simulink model "Torque_Vectoring_Controller_Controls_2018_Test"  (R2017b)
settings: Solver=ode45  StartTime=0.0  StopTime=inf  RelTol=1e-3  EnableMultiTasking=on
InitFcn:
  | clear_close
  | dataCar
  | optParam
  | structSensors
  | structSettings
  | structEstimPar
  | structAero
  | structVariables
  | readFuzzyFile
StartFcn:
  | clear_close
  | dataCar
  | optParam
  | structSensors
  | structSettings
  | structEstimPar
  | structAero
  | structVariables
  | readFuzzyFile
undefined symbols (not defined in the file or in its folder): car, sensors
libraries: CarMaker4SL x21, simulink x11
(part 3 of 4)

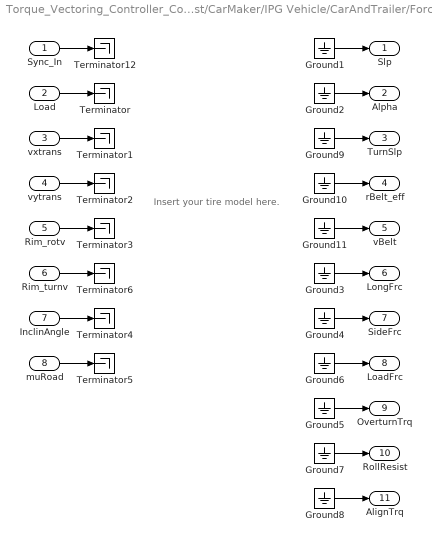
== system Torque_Vectoring_Controller_Controls_2018_Test/CarMaker/IPG Vehicle/CarAndTrailer/Forces/Tires/TireRL ==
  note: Insert your tire model here.
  Sync_In : Inport
  Load : Inport  Port=2
  vxtrans : Inport  Port=3
  vytrans : Inport  Port=4
  Rim_rotv : Inport  Port=5
  Rim_turnv : Inport  Port=6
  InclinAngle : Inport  Port=7
  muRoad : Inport  Port=8
  Ground{1..11} (11 alike) : Ground
  Terminator{,1..6,12} (8 alike) : Terminator
  Slp : Outport
  Alpha : Outport  Port=2
  TurnSlp : Outport  Port=3
  rBelt_eff : Outport  Port=4
  vBelt : Outport  Port=5
  LongFrc : Outport  Port=6
  SideFrc : Outport  Port=7
  LoadFrc : Outport  Port=8
  OverturnTrq : Outport  Port=9
  RollResist : Outport  Port=10
  AlignTrq : Outport  Port=11
  wires:
  Ground11/1 -> vBelt/1
  Ground10/1 -> rBelt_eff/1
  Ground9/1 -> TurnSlp/1
  Rim_turnv/1 -> Terminator6/1
  Sync_In/1 -> Terminator12/1
  Ground2/1 -> Alpha/1
  Ground3/1 -> LongFrc/1
  Ground4/1 -> SideFrc/1
  Ground5/1 -> OverturnTrq/1
  vxtrans/1 -> Terminator1/1
  vytrans/1 -> Terminator2/1
  Rim_rotv/1 -> Terminator3/1
  InclinAngle/1 -> Terminator4/1
  muRoad/1 -> Terminator5/1
  Load/1 -> Terminator/1
  Ground1/1 -> Slp/1
  Ground6/1 -> LoadFrc/1
  Ground7/1 -> RollResist/1
  Ground8/1 -> AlignTrq/1

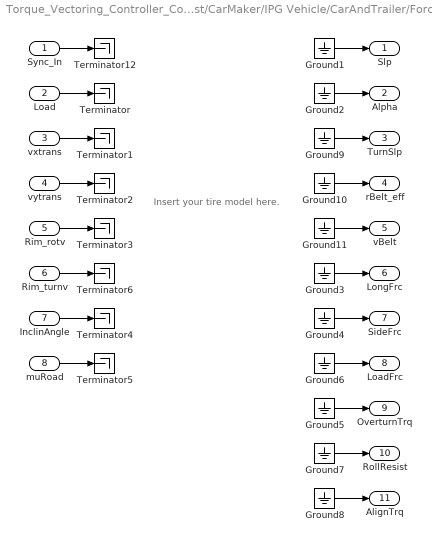
== system Torque_Vectoring_Controller_Controls_2018_Test/CarMaker/IPG Vehicle/CarAndTrailer/Forces/Tires/TireRR ==
  note: Insert your tire model here.
  Sync_In : Inport
  Load : Inport  Port=2
  vxtrans : Inport  Port=3
  vytrans : Inport  Port=4
  Rim_rotv : Inport  Port=5
  Rim_turnv : Inport  Port=6
  InclinAngle : Inport  Port=7
  muRoad : Inport  Port=8
  Ground{1..11} (11 alike) : Ground
  Terminator{,1..6,12} (8 alike) : Terminator
  Slp : Outport
  Alpha : Outport  Port=2
  TurnSlp : Outport  Port=3
  rBelt_eff : Outport  Port=4
  vBelt : Outport  Port=5
  LongFrc : Outport  Port=6
  SideFrc : Outport  Port=7
  LoadFrc : Outport  Port=8
  OverturnTrq : Outport  Port=9
  RollResist : Outport  Port=10
  AlignTrq : Outport  Port=11
  wires:
  Ground11/1 -> vBelt/1
  Ground10/1 -> rBelt_eff/1
  Ground9/1 -> TurnSlp/1
  Rim_turnv/1 -> Terminator6/1
  Sync_In/1 -> Terminator12/1
  Ground2/1 -> Alpha/1
  Ground3/1 -> LongFrc/1
  Ground4/1 -> SideFrc/1
  Ground5/1 -> OverturnTrq/1
  vxtrans/1 -> Terminator1/1
  vytrans/1 -> Terminator2/1
  Rim_rotv/1 -> Terminator3/1
  InclinAngle/1 -> Terminator4/1
  muRoad/1 -> Terminator5/1
  Load/1 -> Terminator/1
  Ground1/1 -> Slp/1
  Ground6/1 -> LoadFrc/1
  Ground7/1 -> RollResist/1
  Ground8/1 -> AlignTrq/1

== matlab function Torque_Vectoring_Controller_Controls_2018_Test/CarMaker/Controls/Control Systems/Traction Control ==
  data: sensors input; Torques output; settings input; estimPar input; torqueDistribution input; slipSet input; car parameter; TiTi2 output; error output; rpmSet output
function [Torques, TiTi2, error, rpmSet] = Traction(sensors, settings, estimPar, torqueDistribution, slipSet, car)

Torquesmin = -car.motor.Tmax;
Torquesmax = car.motor.Tmax;
rpmSetmin = -20000;
rpmSetmax = 20000;

error =[0 0 0 0]';
persistent errorInt; if isempty(errorInt); errorInt=[0 0 0 0]'; end
persistent errorD; if isempty(errorD); errorD=[0 0 0 0]'; end
persistent errorPrev; if isempty(errorPrev); errorPrev=[0 0 0 0]'; end

%persistent wi_prev; if isempty(wi_prev); wi_prev=[0 0 0 0]'; end
%persistent SR_expected; if isempty(SR_expected); SR_expected=zeros(4, 8); end
%persistent wvi_prev; if isempty(wvi_prev); wvi_prev=[0 0 0 0]'; end

persistent TiPrev; if isempty(TiPrev); TiPrev=[0 0 0 0]'; end

persistent errorInt2; if isempty(errorInt2); errorInt2=[0 0 0 0]'; end
persistent Ti; if isempty(Ti); Ti=[0 0 0 0]'; end
persistent Ti2; if isempty(Ti2); Ti2=[0 0 0 0]'; end

rpmSet = [20000;20000;20000;20000];

if settings.TC == 1

    slipRatioTarget = slipSet;
    dist = estimPar.Fzi/sum(estimPar.Fzi);
    
    Kp = 1000*dist*10;
    Ki = 40*dist*1000;
    Kd = 0*dist/100;
    Kv = 1;
    Mu = 1.40;
    
    Kp2 = 20*dist/1000;
    Ki2 = 40*dist/1000;
    
    %normal non linear torque control
    error = slipRatioTarget - estimPar.slip;
    
    errorInt = errorInt + error*car.dt;
    errorInt = min(max(errorInt,-0.001*[1;1;1;1]),0.003*[1;1;1;1]);
    errorD = min(max(errorD*0.1 + 0.9*(error - errorPrev)/car.dt,-25),25);
    lambdaD = Kp.*error + Ki.*errorInt + Kd.*errorD;
    Ti = lambdaD*car.tireInertia*max(estimPar.v,0)^Kv/car.tireRadius + sign(torqueDistribution).*estimPar.Fzi*(Mu)*car.tireRadius;
    Ti = Ti / car.gearRatio;
    
    %optimum seeking
    dFds = dFdsCalculator(estimPar.Fxi,estimPar.slip);
    error2 = dFds - 0;
    errorInt2 = errorInt2 + error2*car.dt;
    errorInt2 = min(max(errorInt2,-500*[1;1;1;1]),500*[1;1;1;1]);
    lambdaD2 = Kp2.*error2 + Ki2.*errorInt2;
    Ti2 = lambdaD2*car.tireInertia*max(estimPar.v,0)^Kv/car.tireRadius + sign(torqueDistribution).*estimPar.Fzi*(car.TC_mu)*car.tireRadius;
    Ti2 = Ti2 / car.gearRatio;
    
    for i=1:4
        if abs(error(i)) < 0.05
            Ti(i) = Ti2(i);
        end
    end
    
    if estimPar.v < 1/3.6
        %Ti = [80 80 180 180]';
        errorInt = [0 0 0 0]';
    end

    if sensors.throttle < 0.1
        errorInt = [0 0 0 0]';
    end
    
    lowerBoundary = TiPrev - 100/car.gearRatio;
    upperBoundary = TiPrev + 100/car.gearRatio;

    Ti = min(max(Ti,lowerBoundary),upperBoundary);
    
    TiPrev = Ti;
    errorPrev = error;
    
    Torques = Ti;
    for i=1:4
        if torqueDistribution(i) > 0
            Torques(i) = max(min(Torques(i),torqueDistribution(i)),0); 
        else
            Torques(i) = min(max(Torques(i),torqueDistribution(i)),0);
        end
    end
    
    
else
    Torques = torqueDistribution;
end

checkTorquemax = find((Torques > car.motor.Tmax)==1); %Limit torques to max torque
Torques(checkTorquemax)=car.motor.Tmax(checkTorquemax);



%wi_prev = sensors.wheelspeed;
%wvi_prev = sensors.wheelspeedi;

TiTi2 = [Ti;Ti2];

Torques = min(max(Torques,Torquesmin),Torquesmax);
rpmSet = min(max(rpmSet,rpmSetmin),rpmSetmax);

end

function [dFds] = dFdsCalculator(Fx,slipRatio)
N = 6;

persistent slipVector, if isempty(slipVector); slipVector = zeros(N,4); end
persistent FxVector, if isempty(FxVector); FxVector = zeros(N,4); end


FxVector(1,:) = Fx;
slipVector(1,:) = slipRatio;

dFds = [0;0;0;0];

for i=1:4
    p1 = polyfit(slipVector(:,i),FxVector(:,i),1);
    p2 = polyfit(FxVector(:,i),slipVector(:,i),1);
    
    rico1 = p1(1);
    rico2 = 1/p2(1);
    
    rico = sign(min(abs(rico1),abs(rico2)))*min(abs(rico1),abs(rico2));

    dFds(i) = max(min(rico,20000),-20000);
end

% shift list one
dummy = FxVector(1:N-1,:);
FxVector = [[0,0,0,0];dummy];
dummy = slipVector(1:N-1,:);
slipVector = [[0,0,0,0];dummy];


end

== matlab function Torque_Vectoring_Controller_Controls_2018_Test/CarMaker/Controls/Vehicle Estimated Parameters/Global model calculation ==
  data: sensors input; F_KF output; States input; H_KF output; y_pred output; yawrate_lin output; beta_lin output; car parameter
function [F_KF, H_KF, y_pred, yawrate_lin, beta_lin] = global_model(sensors, States, car)

global vy_g psi_dot_g vx_g Cf_g Cr_g vy_lin psi_dot_lin

if isempty(vy_g) == 1 && isempty(psi_dot_g) == 1 && isempty(vx_g) == 1 ...
        && isempty(Cf_g) == 1 && isempty(Cr_g) == 1 
    States.vy_g = 0;
    States.psi_dot_g = 0;
    States.vx_g = 0;
    States.Cf_g = 0;
    States.Cr_g = 0;
    
else 
    
    States.vy_g = vy_g;
    States.psi_dot_g = psi_dot_g;
    States.vx_g = vx_g;
    States.Cf_g = Cf_g;
    States.Cr_g = Cr_g;
    delta = (sensors.wheelAngles(1)+sensors.wheelAngles(2))/2;
    
    %% Calculating F_KF %%
    
    F_vy = [-(2*(States.Cf_g+States.Cr_g))/(car.mass*States.vx_g),...
        -((2*(States.Cf_g*car.lf-States.Cr_g*car.lr))/(car.mass*States.vx_g))+States.vx_g,...
        (((2*(States.Cf_g+States.Cr_g))/(car.mass*States.vx_g^2))*States.vy_g)+...
        (((2*(States.Cf_g*car.lf-States.Cr_g*car.lr))/(car.mass*States.vx_g^2))*States.psi_dot_g)-States.psi_dot_g,...
        (-2/(car.mass*States.vx_g))*(States.vy_g+car.lf*States.psi_dot_g)+(2*delta/car.mass),...
        (-2/(car.mass*States.vx_g))*(States.vy_g-car.lr*States.psi_dot_g)];
    
    F_psi_dot = [-(2*(States.Cf_g*car.lf-States.Cr_g*car.lr))/(car.yawInertia*States.vx_g),...
        -((2*(States.Cf_g*car.lf^2+States.Cr_g*car.lr^2))/(car.yawInertia*States.vx_g)),...
        (((2*(States.Cf_g*car.lf-States.Cr_g*car.lr))/(car.yawInertia*States.vx_g^2))*States.vy_g)+...
        (((2*(States.Cf_g*car.lf^2+States.Cr_g*car.lr^2))/(car.yawInertia*States.vx_g^2))*States.psi_dot_g),...
        (-2*car.lf/(car.yawInertia*States.vx_g))*(States.vy_g+car.lf*States.psi_dot_g)+(2*delta*car.lf/car.yawInertia),...
        (2*car.lr/(car.yawInertia*States.vx_g))*(States.vy_g-car.lr*States.psi_dot_g)];
    
    F_vx = [States.psi_dot_g, States.vy_g,0,0,0];
    
    F_Cf = [0,0,0,0,0];
    
    F_Cr = [0,0,0,0,0];
    
    F_KF = [F_vy;F_psi_dot;F_vx;F_Cf;F_Cr];
    
    %% Calculation vy_lin and beta_lin %% Gelineariseerd, hier kan eventueel ook
    % ode45 voor gebruikt worden.
    
   A_1 = (-2*(car.Cf_lin + car.Cr_lin))/(car.mass*States.vx_g);
   A_2 = -((2*(car.Cf_lin*car.lf - car.Cr_lin*car.lr))/(car.mass*States.vx_g))+States.vx_g;
   A_3 = -(2*(car.Cf_lin*car.lf - car.Cr_lin*car.lr))/(car.yawInertia*States.vx_g);
   A_4 = (-2*(car.Cf_lin*car.lf^2 + car.Cr_lin*car.lr^2))/(car.yawInertia*States.vx_g);
   
   B_1 = (2*car.Cf_lin*delta)/(car.mass);
   B_2 = (2*car.Cf_lin*car.lf*delta)/(car.yawInertia);
      
   A = [1+A_1*car.dt, A_2*car.dt; A_3*car.dt 1+A_4*car.dt];
   B = [B_1; B_2];
   
   
   lin_var = A*[vy_lin;psi_dot_lin] + B;
   vy_lin = lin_var(1);
   psi_dot_lin = lin_var(2);
   yawrate_lin =  psi_dot_lin;
   beta_lin = vy_lin/(States.vx);
    
    %% Calculation H_KF %%
    
    H_psi_dot = [0, 1, 0, 0,0];
    
    H_ay = [-(2*(States.Cf_g+States.Cr_g))/(car.mass*States.vx_g),...
        -((2*(States.Cf_g*car.lf-States.Cr_g*car.lr))/(car.mass*States.vx_g)),...
        (((2*(States.Cf_g+States.Cr_g))/(car.mass*States.vx_g^2))*States.vy_g)+...
        (((2*(States.Cf_g*car.lf-States.Cr_g*car.lr))/(car.mass*States.vx_g^2))*States.psi_dot_g),...
        (-2/(car.mass*States.vx_g))*(States.vy_g+car.lf*States.psi_dot_g)+(2*delta/car.mass),...
        (-2/(car.mass*States.vx_g))*(States.vy_g-car.lr*States.psi_dot_g)];
    
    H_vxfl = [sin(sensors.wheelAngles(1)),  -(car.tf/2)*cos(sensors.wheelAngles(1))+car.lf*sin(sensors.wheelAngles(1)), cos(sensors.wheelAngles(1)), 0, 0];
    
    H_vxfr = [sin(sensors.wheelAngles(2)), (car.tf/2)*cos(sensors.wheelAngles(2))+car.lf*sin(sensors.wheelAngles(2)), cos(sensors.wheelAngles(2)),  0, 0];
    
    H_vxrl = [0, -(car.tr/2), 1, 0, 0];
    
    H_vxrr = [0, (car.tr/2), 1, 0, 0];
    
    H_beta_lin = [0,0,-(vy_lin/States.vx_g^2),0,0]; %afgeleide naar vx herplaatst, die naar vy = 0?
    
    H_KF = [H_psi_dot;H_ay;H_vxfl;H_vxfr;H_vxrl;H_vxrr; H_beta_lin];

    %% Calculation of y_pred
    
    y_pred.yawrate = States.psi_dot_g;
    
    y_pred.ay = (-2*(States.Cf_g+States.Cr_g)/(car.mass*States.vx_g))*(States.vy) - ...
        (2*(States.Cf_g*car.lf-States.Cr_g*car.lr)/(car.mass*States.vx_g))*(States.psi_dot_g) +... % - teken aangepast naar vgl (7) uit van Aalst
        (2*States.Cf_g*delta/car.mass);
    
    y_pred.vxfl = (States.vx_g - States.psi_dot_g*(car.tf/2))*cos(sensors.wheelAngles(1)) + ...
        (States.vy_g + States.psi_dot_g*(car.lf))*sin(sensors.wheelAngles(1));
    
    y_pred.vxfr = (States.vx_g + States.psi_dot_g*(car.tf/2))*cos(sensors.wheelAngles(2)) + ...
        (States.vy_g + States.psi_dot_g*(car.lf))*sin(sensors.wheelAngles(2));
    
    y_pred.vxrl = (States.vx_g - States.psi_dot_g*(car.tr/2));
    
    y_pred.vxrr = (States.vx_g + States.psi_dot_g*(car.tr/2));
    
    y_pred.beta_lin = (vy_lin)/(States.vx);
    
end
end

== matlab function Torque_Vectoring_Controller_Controls_2018_Test/CarMaker/Controls/Control Systems/Yaw Rate Control ==
  data: sensors input; Mz output; settings input; estimPar input; car parameter; error output; actions output; rref output
function [Mz,error,actions,rref]= yawRateControl(sensors, settings, estimPar, car)
%Function that controls the moment around the z-axis
%INPUTS:
%OUTPUT: Moment of the car around Z-axis [Nm]

Mz = 0;
Mz_temp = 0;
rref = estimPar.rref;
error = 0;


wheelAngle = (sensors.wheelAngles(1)+sensors.wheelAngles(2))/2;

%For analyzation
P_Action = 0;
I_Action = 0;
D_Action = 0;

steeringWheel_Action = 0;
yawRate_Action = 0;

persistent Mz_memory; if isempty(Mz_memory); Mz_memory = 0; end
persistent errorInt; if isempty(errorInt); errorInt = 0; end
persistent errorDev; if isempty(errorDev); errorDev = 0; end
persistent prevError; if isempty(prevError); prevError = 0; end
persistent prevWheelAngle; if isempty(prevWheelAngle); prevWheelAngle = 0; end
persistent prevRref; if isempty(prevRref); prevRref = 0; end

%if settings.YRCMode == 1
error = estimPar.rref - sensors.yawRate;
errorInt = errorInt + error*car.dt;
errorInt = min(max(errorInt,-car.YRC.intLimit),car.YRC.intLimit);
errorDev = (error - prevError)/car.dt;
wheelAngleFF = wheelAngle;


velocityGain = min(max(1 - (estimPar.v - car.YRC.changeVelocity)*car.YRC.slope,0),1);

Mz_temp = (car.YRC.Kp*error + car.YRC.Ki*errorInt + car.YRC.Kd*errorDev...
    +car.YRC.Ks*wheelAngleFF)*velocityGain;
Mz_temp = max(min(Mz_temp,car.YRC.maxValue),-car.YRC.maxValue);
Mz_memory=Mz_memory+Mz_temp;

P_Action = car.YRC.Kp*error;
I_Action = car.YRC.Ki*errorInt;
D_Action = car.YRC.Kd*errorDev;
steeringWheel_Action = car.YRC.Ks*wheelAngle;
yawRate_Action = car.YRC.Kr*estimPar.rref;

actions = [P_Action;I_Action;D_Action;steeringWheel_Action;yawRate_Action];
prevError = error;
prevWheelAngle = wheelAngle;
prevRref = estimPar.rref;
%end


% if settings.YRCMode == 2
%     error = estimPar.rref - sensors.yawRate;
%     integral = integral + error*car.dt;
%     derivative = (error - prevError)/car.dt;
%
%     Mz_temp = car.YRC.Kp*error + car.YRC.Ki*integral + car.YRC.Kd*derivative...
%         +car.YRC.Ks*wheelAngle + car.YRC.Kr*estimPar.rref;
%     Mz_temp = max(min(Mz_temp,car.YRC.maxValue),-car.YRC.maxValue);
%
%     prevError = error;
% end





%YRC enabled
if settings.YRC ==1
    Mz = Mz_memory;
    
    %YRC disabled
else
    Mz = 0;
end

if car.YRC.minV > estimPar.v
    Mz = 0; %if speed is too low, don't activate yaw rate control
    errorInt = 0;
    prevError = 0;
end



rref=estimPar.rref;

Mz = min(max(Mz,-car.MzMax),car.MzMax); % set limits to maximum sent out Mz

== matlab function Torque_Vectoring_Controller_Controls_2018_Test/CarMaker/Controls/Controller Settings/Controller Settings ==
  data: settings output Bus: settingBus; sensors input; variables output Bus: variableBus
function [settings,variables] = settingController(sensors)

%% Settings

%Afblijven van dit, dit is de default instelling
velocityEstimation_Temp = 0;
YRCMode_Temp = 0;
torqueMode_Temp = 0;
YRC_Temp = 0;
TC_Temp = 0;
unlimitedFx_Temp = 0;
effEstimation_Temp = 0;


%if sensors.knob1 == 1
    YRC_Temp = 1;
%end

%if sensors.knob1 == 1
    torqueMode_Temp = 2; %Change distributor mode
%end

%if sensors.knob2 == 1
    YRCMode_Temp = 1;
    TC_Temp = 0;
    unlimitedFx_Temp = 0;
    TV_bypass_Temp = 0;
%end
velocityEstimation_Temp = 1;
%if sensors.knob2 == 2
    %YRCMode_Temp = 2;
%end

effEstimation_Temp = 2;

%% Variables
TD_percentage_Temp = 1;


%% Declaration Settings

settings.velocityEstimation = velocityEstimation_Temp;
settings.torqueMode = torqueMode_Temp;
settings.YRC = YRC_Temp;
settings.YRCMode = YRCMode_Temp;
settings.distributorMode = 0;

settings.Fsens = 100; %value between 0 and 100
% 100 --> Fdes is really important
% 0 --> Mdes is really important

settings.Fxsens = 1;

settings.TC = TC_Temp;
settings.unlimitedFx = unlimitedFx_Temp;
settings.TV_bypass = TV_bypass_Temp;
settings.effEstimation = effEstimation_Temp;

%% Declaration Variables
variables.TD_percentage = TD_percentage_Temp;

== matlab function Torque_Vectoring_Controller_Controls_2018_Test/CarMaker/Controls/Vehicle Estimated Parameters/Scopes/States decomposition ==
  data: States input; vy output; psi_dot output; vx output; Cf output; Cr output
function [vy,psi_dot,vx,Cf,Cr] = state_decomp(States)

vy = States.vy_g;
psi_dot = States.psi_dot_g;
vx = States.vx_g;
Cf = States.Cf_g;
Cr = States.Cr_g;

== matlab function Torque_Vectoring_Controller_Controls_2018_Test/CarMaker/Controls/Vehicle Estimated Parameters/Scopes/alpha decomposition ==
  data: alpha input; alpha_f output; alpha_r output
function [alpha_f, alpha_r] = alpha_decomp(alpha)

alpha_f = alpha.f;
alpha_r = alpha.r;

end

== matlab function Torque_Vectoring_Controller_Controls_2018_Test/CarMaker/Controls/Vehicle Estimated Parameters/Velocity and alpha decomposition ==
  data: States input; vx_wheels output; vy_wheels output; alpha_wheels output; sensors parameter; car parameter
function [vx_wheels, vy_wheels, alpha_wheels] = v_alpha_decomp(States, sensors, car)

%% Calculation vx on each independant wheel %%

vx_wheels.fl = (States.vx_g - States.psi_dot_g*(car.tf/2))*cos(sensors.wheelAngles(1)) + ...
        States.psi_dot_g*(car.lf)*sin(sensors.wheelAngles(1));
    
vx_wheels.fr = (States.vx_g + States.psi_dot_g*(car.tf/2))*cos(sensors.wheelAngles(2)) + ...
        States.psi_dot_g*(car.lf)*sin(sensors.wheelAngles(2));
    
vx_wheels.rl = (States.vx_g - States.psi_dot_g*(car.tr/2));
    
vx_wheels.rr = (States.vx_g + States.psi_dot_g*(car.tr/2));

%% Calculation vy on each independant wheel %%

vy_wheels.fl = (States.vy_g + States.psi_dot_g*(car.lf))*cos(sensors.wheelAngles(1)) + ...
        States.psi_dot_g*(car.tf/2)*sin(sensors.wheelAngles(1));
    
vy_wheels.fr = (States.vy_g - States.psi_dot_g*(car.tf/2))*sin(sensors.wheelAngles(2)) + ...
        States.psi_dot_g*(car.lf)*cos(sensors.wheelAngles(2));
    
vy_wheels.rl = (States.vy_g - States.psi_dot_g*(car.lr));
    
vy_wheels.rr = (States.vy_g - States.psi_dot_g*(car.lr));

%% Calculation alpha's on each independant wheel %%

alpha_wheels.fl = atan2(vy_wheels.fl,vx_wheels.fl);
alpha_wheels.fr = atan2(vy_wheels.fr,vx_wheels.fr);
alpha_wheels.rl = atan2(vy_wheels.rl,vx_wheels.rl);
alpha_wheels.rr = atan2(vy_wheels.rr,vx_wheels.rr);

== matlab function Torque_Vectoring_Controller_Controls_2018_Test/CarMaker/Controls/Control Systems/Distributor/MATLAB Function ==
  data: sensors input; torqueDistribution output; settings input; estimPar input; car parameter; variables input; Mz input; slipSet output; Fdes output; sumFx output; Fxmax output; Fxmaxsum output; Fx output; Fdes input
function [torqueDistribution, slipSet,Fdes,sumFx,Fxmax,Fxmaxsum, Fx]= TorqueDistributor(sensors,settings, estimPar, car, variables, Mz, Fdes)
%,Fdes,sumFx,Fxmax,Fxmaxsum

torqueDistribution = [0;0;0;0];
slipSet = [0;0;0;0];


sumFx=0;
Fxmax=[0;0;0;0];
Fxmaxsum=0;
Fx=[0;0;0;0];
if settings.torqueMode == 1
    
    dT =  0.25*Mz/(car.tw*0.5)*car.tireRadius;
    torqueDistribution = car.motor.Tmax*variables.TD_percentage*sensors.throttle;
    torqueDistribution = torqueDistribution + [-1; 1; -1; 1]*dT;
    
    for i=1:4
        if torqueDistribution(i) > 0
            slipSet(i) = car.TC.slipSetAcc;
        else
            slipSet(i) = car.TC.slipSetBrake;
        end
    end
    
    
end



%Test torque mode: only Fx, no steeringAngle

if settings.torqueMode == 2
    

    
    Fxmax = [0;0;0;0];
    %minForce = 2*car.Cd*car.AFront*0.5*car.rhoAir*estimPar.v*estimPar.v*0.25; %2* of niet? en met Cd?
    minForce = 0;
    %FyReduceFactor = 0.1;
    %Fxmax = (max((estimPar.mu .* estimPar.Fzi).^2-FyReduceFactor*estimPar.Fyi.^2,0).^0.5); %Kamm's circle
    
    
    
    Fxmax = estimPar.mu.*estimPar.Fzi;
    
    Fxmax = max(Fxmax,minForce);
    motorSpeed = min(max(sensors.wheelspeed.*car.gearRatio,0),20000);
    FxmaxMax = [car.FxmaxMax(round(motorSpeed(1)+1));...
        car.FxmaxMax(round(motorSpeed(2)+1));...
        car.FxmaxMax(round(motorSpeed(3)+1));...
        car.FxmaxMax(round(motorSpeed(4)+1))];  %make sure the max torque of the motor isn't surpassed

%     x = 0:10:22000; y = [0 .15 1.12 2.36 2.36 1.46 .49 .06 0];
%     cs = spline(x,[0 y 0]);
%     xx = linspace(-4,4,101);
%     plot(x,y,'o',xx,ppval(cs,xx),'-');
    
    checkFxmax = find((Fxmax > FxmaxMax)==1);
    Fxmax(checkFxmax)=FxmaxMax(checkFxmax);
    
    if settings.unlimitedFx == 1  %Surpass the tire grip limits in case if the driver feels to restricted with this.
        Fxmax = FxmaxMax;
    end
    
    Fxmaxsum = sum(Fxmax);
    Fxmin = -Fxmax;
    
    Fx = [0;0;0;0];
    
    
    Fx = Distributor(settings, car, Mz, Fdes, Fxmax, Fxmin);
    
    torqueDistribution = car.tireRadius*Fx; %torque of motor, NOT of wheels (as IPG expects this as input)
    
    for i=1:4
        if torqueDistribution(i) > 0
            slipSet(i) = car.TC.slipSetAcc;
        else
            slipSet(i) = car.TC.slipSetBrake;
        end
    end
    
    sumFx = sum(Fx);
end



torqueDistribution = min(max(torqueDistribution,-car.motor.Tmax),car.motor.Tmax); % dees nog ifv motorkarakteristiek
end

== matlab function Torque_Vectoring_Controller_Controls_2018_Test/CarMaker/Controls/Bypass/MATLAB Function ==
  data: settings input; torqueBypass output; sensors input; rpmBypass output; car parameter
function [torqueBypass,rpmBypass]= fcn(settings, sensors, car)
PmaxTyre = car.Pmax_bypass*0.25;
rad2rpm = 30/pi;


safetyFactor = 0.5;
torqueBypass = car.motor.Tmax*safetyFactor*car.gearRatio*sensors.throttle;

if sensors.throttle > 0
    rpmBypass = car.motor.rpmMax;
else
    rpmBypass = [0;0;0;0];
end

%% Power limiter
limit = PmaxTyre./max(sensors.wheelspeed,1);
torqueBypass = max(min(torqueBypass,limit),-limit);

== matlab function Torque_Vectoring_Controller_Controls_2018_Test/CarMaker/Controls/Vehicle Estimated Parameters/Scopes/Longitudinal velocity decomposition ==
  data: vx_wheels input; vx_fl output; vx_fr output; vx_rl output; vx_rr output
function [vx_fl, vx_fr, vx_rl, vx_rr] = long_vel_decomp(vx_wheels)

vx_fl = vx_wheels.fl;
vx_fr = vx_wheels.fr;
vx_rl = vx_wheels.rl;
vx_rr = vx_wheels.rr;

end

== matlab function Torque_Vectoring_Controller_Controls_2018_Test/CarMaker/Controls/Tire model//friction coefficient estimation/MATLAB Function ==
  data: mu input; estimParExtended output; estimPar input
function estimParExtended  = estimParExtension(mu, estimPar)

estimParExtended.vy_g = estimPar.vy_g;
estimParExtended.psi_dot_g = estimPar.psi_dot_g;
estimParExtended.vx_g = estimPar.vx_g;
estimParExtended.Cf_g = estimPar.Cf_g;
estimParExtended.Cr_g = estimPar.Cr_g;
estimParExtended.Fzi=estimPar.Fzi;
estimParExtended.Fxi=estimPar.Fxi;
estimParExtended.Fyi=estimPar.Fyi;
estimParExtended.alpha_f = estimPar.alpha.f;
estimParExtended.alpha_r = estimPar.alpha.r;
estimParExtended.eff = estimPar.eff;
estimParExtended.mu = mu;
estimParExtended.rref = estimPar.rref;

== matlab function Torque_Vectoring_Controller_Controls_2018_Test/CarMaker/IPG Feedback/Subsystem/MATLAB Function ==
  data: Wheelspeed_Max input; T_mot output; Wheelspeed_Sens input; Treq input
function T_mot = SpeedLimit(Wheelspeed_Max,Wheelspeed_Sens,Treq)
%Speed limiter for IPG Carmaker
if Wheelspeed_Sens>= Wheelspeed_Max
    T_mot=0;
else
    T_mot=Treq;
end

== matlab function Torque_Vectoring_Controller_Controls_2018_Test/CarMaker/Controls/Tire model//friction coefficient estimation/Magic_Tire_Param_Scope ==
  data: Magic_tire_param input; MTF_tire_model_front_x output; estimParBus input; Fzi input; MTF_tire_model_front_y output; MTF_tire_model_rear_x output; MTF_tire_model_rear_y output
function [MTF_tire_model_front_x, MTF_tire_model_front_y,MTF_tire_model_rear_x,...
    MTF_tire_model_rear_y] = Scope_Magig_tire(Magic_tire_param, estimParBus, Fzi)

MTF_tire_model_front_x = (Fzi(1)*Magic_tire_param.front_x(3))*sin(Magic_tire_param.front_x(2)*...
    atan(Magic_tire_param.front_x(1)*(1-Magic_tire_param.front_x(4))*estimParBus.alpha_f +...
    atan(Magic_tire_param.front_x(1)*estimParBus.alpha_f)));

MTF_tire_model_front_y = (Fzi(2)*Magic_tire_param.front_y(3))*sin(Magic_tire_param.front_y(2)*...
    atan(Magic_tire_param.front_y(1)*(1-Magic_tire_param.front_y(4))*estimParBus.alpha_r +...
    atan(Magic_tire_param.front_y(1)*estimParBus.alpha_r)));

MTF_tire_model_rear_x = (Fzi(3)*Magic_tire_param.rear_x(3))*sin(Magic_tire_param.rear_x(2)*...
    atan(Magic_tire_param.rear_x(1)*(1-Magic_tire_param.rear_x(4))*estimParBus.alpha_f +...
    atan(Magic_tire_param.rear_x(1)*estimParBus.alpha_f)));

MTF_tire_model_rear_y = (Fzi(4)*Magic_tire_param.rear_y(3))*sin(Magic_tire_param.rear_y(2)*...
    atan(Magic_tire_param.rear_y(1)*(1-Magic_tire_param.rear_y(4))*estimParBus.alpha_r +...
    atan(Magic_tire_param.rear_y(1)*estimParBus.alpha_r)));

end

== matlab function Torque_Vectoring_Controller_Controls_2018_Test/CarMaker/Controls/Vehicle Estimated Parameters/Scopes/Lateral velocity decomposition1 ==
  data: vy_wheels input; vy_fl output; vy_fr output; vy_rl output; vy_rr output
function [vy_fl, vy_fr, vy_rl, vy_rr] = lat_vel_decomp(vy_wheels)

vy_fl = vy_wheels.fl;
vy_fr = vy_wheels.fr;
vy_rl = vy_wheels.rl;
vy_rr = vy_wheels.rr;

end

== matlab function Torque_Vectoring_Controller_Controls_2018_Test/CarMaker/Controls/Vehicle Estimated Parameters/Scopes/Slip angle decomposition1 ==
  data: alpha_wheels input; alpha_fl output; alpha_fr output; alpha_rl output; alpha_rr output
function [alpha_fl, alpha_fr, alpha_rl, alpha_rr] = alpha_decomp(alpha_wheels)

alpha_fl = alpha_wheels.fl;
alpha_fr = alpha_wheels.fr;
alpha_rl = alpha_wheels.rl;
alpha_rr = alpha_wheels.rr;

end

== matlab function Torque_Vectoring_Controller_Controls_2018_Test/CarMaker/IPG Feedback/Subsystem/MATLAB Function1 ==
  data: Wheelspeed_Max input; T_mot output; Wheelspeed_Sens input; Treq input
function T_mot = SpeedLimit(Wheelspeed_Max,Wheelspeed_Sens,Treq)
%Speed limiter for IPG Carmaker
if Wheelspeed_Sens>= Wheelspeed_Max
    T_mot=0;
else
    T_mot=Treq;
end

== matlab function Torque_Vectoring_Controller_Controls_2018_Test/CarMaker/IPG Feedback/Subsystem/MATLAB Function2 ==
  data: Wheelspeed_Max input; T_mot output; Wheelspeed_Sens input; Treq input
function T_mot = SpeedLimit(Wheelspeed_Max,Wheelspeed_Sens,Treq)
%Speed limiter for IPG Carmaker
if Wheelspeed_Sens>= Wheelspeed_Max
    T_mot=0;
else
    T_mot=Treq;
end

== matlab function Torque_Vectoring_Controller_Controls_2018_Test/CarMaker/IPG Feedback/Subsystem/MATLAB Function3 ==
  data: Wheelspeed_Max input; T_mot output; Wheelspeed_Sens input; Treq input
function T_mot = SpeedLimit(Wheelspeed_Max,Wheelspeed_Sens,Treq)
%Speed limiter for IPG Carmaker
if Wheelspeed_Sens>= Wheelspeed_Max
    T_mot=0;
else
    T_mot=Treq;
end

== matlab function Torque_Vectoring_Controller_Controls_2018_Test/CarMaker/Controls/Subsystem/MATLAB Function ==
  data: torqueController input; torques output; rpmController input; torqueBypass input; rpmBypass input; rpmRef output; settings input
function [torques,rpmRef]= fcn(torqueController,rpmController,torqueBypass,rpmBypass,settings)
%#codegen

torques = [0;0;0;0];
rpmRef = [0;0;0;0];

if settings.TV_bypass == 0

    torques = torqueController;
    rpmRef = rpmController;

elseif settings.TV_bypass == 1
    
    torques = torqueBypass;
    rpmRef = rpmBypass;
end

== matlab function Torque_Vectoring_Controller_Controls_2018_Test/CarMaker/Controls/Control Systems/Distributor/Torque//Brake analyzer/MATLAB Function1 ==
  data: sensors input; Fdes output; settings input; estimPar input; variables input; car parameter
function Fdes = Fdes(sensors, settings, estimPar, variables,car)
    


%Fdes = 11*4* min(car.motor.Tmax)*variables.TD_percentage*sensors.throttle/car.tireRadius;
    %if sensors.throttle > 0
    %Fdes = sum(car.motor.Tmax)*variables.TD_percentage*sensors.throttle/car.tireRadius; % *4 because four motors
    %Fdes = Fdes*car.gearRatio;
    
    Fdes = sum(sensors.throttle*1.5*estimPar.mu*(car.mass*car.g + 0.5*car.rhoAir*estimPar.v*estimPar.v*car.Cl*car.AFront));
    
    if sensors.brake > 0
        Fdes = -sum(car.motor.Tmax)*variables.TD_percentage*sensors.brake/car.tireRadius;
        Fdes = Fdes*car.gearRatio;
    end
    %Fdes= 5000;
    
    %end
    %     Fdes = Fdes*1;
    %     Fdes = 800;
    
    %     Fdes = sensors.throttle*mean(estimPar.mu)*(car.mass*car.g + 0.5*car.rhoAir*estimPar.v*estimPar.v*car.Cl*car.AFront );
    %     Fdes = Fdes;
    

end

== matlab function Torque_Vectoring_Controller_Controls_2018_Test/CarMaker/Controls/Control Systems/Power Checker/Power checker ==
  data: sensors input; settings input; estimPar input; UncheckedTorque input; CheckedTorque output; car parameter; P_mech output; maxMechPower output; power2beReduced output; part2beReduced output; CheckedP_mech output
function [CheckedTorque,P_mech,maxMechPower,power2beReduced,part2beReduced,CheckedP_mech]= fcn(sensors, settings,estimPar, UncheckedTorque, car)

%% Power limiter according to FS rules

P_mech = sum(UncheckedTorque.*sensors.wheelspeed*car.gearRatio); %[Nm*rad/s][W]

maxMechPower = (car.Pmax - car.PC.safetyMargin)*estimPar.eff;
power2beReduced = 0;

if P_mech > maxMechPower
    power2beReduced = P_mech - maxMechPower;
end

if abs(P_mech) > 0.1
    part2beReduced = power2beReduced/P_mech;
else
    part2beReduced = 0;
end

CheckedTorque = UncheckedTorque*max(min((1 - part2beReduced),1),0);
CheckedP_mech = sum(CheckedTorque.*sensors.wheelspeed*car.gearRatio); %[Nm*rad/s][W]

== matlab function Torque_Vectoring_Controller_Controls_2018_Test/CarMaker/Controls/Vehicle Estimated Parameters/Wheel speed calculation ==
  data: sensors input; beta_lin input; y_meas output; car parameter
function y_meas  = wheelspeedcalc(sensors, beta_lin, car)

yaw_rate = sensors.yawRate;
ay = sensors.accy;
vxfl = sensors.wheelspeed(1)*car.tireRadius;
vxfr = sensors.wheelspeed(2)*car.tireRadius;
vxrl = sensors.wheelspeed(3)*car.tireRadius;
vxrr = sensors.wheelspeed(4)*car.tireRadius;

y_meas = [yaw_rate ay vxfl vxfr vxrl vxrr beta_lin];

== matlab function Torque_Vectoring_Controller_Controls_2018_Test/CarMaker/Vehicle Sensors/Sensors ==
  data: ax input; sensors output Bus: sensorBus size=1; ay input; wheelspeed_FL input; wheelspeed_FR input; wheelspeed_RL input; wheelspeed_RR input; yawRate input; steeringAngle input; steerAngleFL input; steerAngleFR input; throttle input; brake input; torqueFL input; torqueFR input; torqueRL input; torqueRR input; ax_error input; ay_error input; yawRate_error input; knob1 input; knob2 input; P_elec_FL input; P_elec_FR input; P_elec_RL input; P_elec_RR input
function sensors = sensors(ax,ay,wheelspeed_FL,wheelspeed_FR,wheelspeed_RL,wheelspeed_RR,yawRate,steeringAngle,steerAngleFL,steerAngleFR, throttle,brake,torqueFL,torqueFR,torqueRL,torqueRR,ax_error,ay_error,yawRate_error,knob1,knob2,P_elec_FL,P_elec_FR,P_elec_RL,P_elec_RR)

sensors.ax = ax;
sensors.ay = ay;
sensors.wheelspeed = [wheelspeed_FL;wheelspeed_FR;wheelspeed_RL;wheelspeed_RR];
sensors.yawRate = yawRate;
sensors.steerAngle = steeringAngle;
sensors.wheelAngles = [steerAngleFL;steerAngleFR;0;0];
sensors.throttle = throttle;
sensors.brake= brake;
sensors.torque = [torqueFL;torqueFR;torqueRL;torqueRR];
sensors.ax_error = ax_error;
sensors.ay_error = ay_error;
sensors.yawRate_error = yawRate_error;
sensors.knob1 = knob1;
sensors.knob2 = knob2;
sensors.P_elec = sum([P_elec_FL;P_elec_FR;P_elec_RL;P_elec_RR]);

== matlab function Torque_Vectoring_Controller_Controls_2018_Test/CarMaker/Controls/Vehicle Estimated Parameters/Extended Kalman Filter ==
  data: F_KF input; States output; H_KF input; y_meas input; y_pred input; R_beta_lin input; Q_Cy input; sensors input; P_est input; P_est output
function [States, P_est]  = EKF(F_KF,H_KF,y_meas, y_pred, R_beta_lin, Q_Cy, sensors, P_est)
 
 %% Initialization of global variables %%
 
global vy_g psi_dot_g vx_g Cf_g Cr_g P_est_glob

delta = (sensors.wheelAngles(1)+sensors.wheelAngles(2))/2;
 %% Calculation partitioned F-matrix %%
F = F_KF;
 
 %% Calculation partitioned H-matrix %%
H = H_KF;

% ============================== Parameters ===============================
% number of observable states
n_xo = 3;
% number of unobservable states
n_xu = 2;
% total number of states
n_x = n_xo + n_xu;
% number of system inputs
n_u = 2;
% number of measurements
n_y = 7;
% covariance of modeled process noise

Q_Cyf = Q_Cy;
Q_Cyr = Q_Cy;
Q_vy = 1*10^(-6);
Q_psi_dot = 1*10^(-6);
Q_vx = 1*10^(-4);

Q_oo = [Q_vy, 0, 0;
    0, Q_psi_dot, 0;
    0, 0, Q_vx];

Q_uu = [Q_Cyf, 0;
     0, Q_Cyr];
 
Q_model = [Q_vy, 0, 0, 0, 0;
    0, Q_psi_dot, 0, 0, 0;
    0, 0, Q_vx, 0, 0;
    0, 0, 0, Q_Cyf, 0;
    0, 0, 0, 0, Q_Cyr];

% covariance of measurement noise

R_psi_dot = 2.4*10^(-7);
R_ay = 2.5*10^(-3);
R_vxfl = 1*10^(-5);
R_vxfr = 1*10^(-5);
R_vxrl = 1*10^(-5);
R_vxrr = 1*10^(-5);
R_beta = R_beta_lin;
R_model = [R_psi_dot, 0, 0, 0, 0, 0, 0;
    0, R_ay, 0, 0, 0, 0, 0;
    0, 0, R_vxfl, 0, 0, 0, 0;
    0, 0, 0, R_vxfr, 0, 0, 0;
    0, 0, 0, 0, R_vxrl, 0, 0;
    0, 0, 0, 0, 0, R_vxrr, 0;
    0, 0, 0, 0, 0, 0, R_beta];
% covariance of simulated process noise
Q_sim = [Q_vy, 0, 0, 0, 0;
    0, Q_psi_dot, 0, 0, 0;
    0, 0, Q_vx, 0, 0;
    0, 0, 0, Q_Cyf, 0;
    0, 0, 0, 0, Q_Cyr];
% covariance of simulated measurement noise
R_sim = [R_psi_dot, 0, 0, 0, 0, 0, 0;
    0, R_ay, 0, 0, 0, 0, 0;
    0, 0, R_vxfl, 0, 0, 0, 0;
    0, 0, 0, R_vxfr, 0, 0, 0;
    0, 0, 0, 0, R_vxrl, 0, 0;
    0, 0, 0, 0, 0, R_vxrr, 0;
    0, 0, 0, 0, 0, 0, R_beta];
% initial state
x0 = [0; 0; 0; car.Cf_lin; car.Cr_lin];
% initial state estimate
% x_est0 = [0; 0; 0; car.Cf_lin; car.Cr_lin];
% feedback values
% kx = 0.1;
% ky = 0.1;
% kt = 0.1;

% ==================== Simulation Preparation ===========================

if isempty(P_est_glob) == 1
    states = x_0;
    P_est= eye(n_x)*10^(-4);
    
else
    states = [vy_g, psi_dot_g, vx_g, Cf_g, Cr_g];
    
end
       
inputs_EKF = [delta; sensors.ax];

P_est_pre_tot = zeros(n_x, n_x);

P_est_post_tot = zeros(n_x, n_x);


% feedback matrix
% K = [kx,  0,  0;
%       0, ky, kt];


% ==================== Kalman prediction step ===========================

states = f_est(states, inputs_EKF, car.dt);

P_est_pre = F*P_est*F^(-1)+Q_model;

%P_est_pre_oo = A*P_est_post(:,:,i-1)*A' + Q_mod;
%      P_est(:,:,i) = A*P_est(:,:,i-1)*A';

% ==================== Kalman correction step ===========================

nu = y_meas - y_pred;
%      nu(:,i) = y(:,i) - h(x_est(:,i));
S = H*P_est_pre*H' + R_model;
%      S(:,:,i) = C*P_est(:,:,i)*C';
K = P_est_pre*H'/S;

states = states + K*nu;
P_est_post = (eye(n_x)-K*H)*P_est_pre;

States.vy_g = states(1);
States.psi_dot_g = states(2);
States.vx_g = states(3);
States.Cf_g = states(4);
States.Cr_g = states(5);

P_est = P_est_post;
P_est_glob = P_est;

% %     Control law
% u(:,i) = u_ref(:,i);
% %     err_loc(:,i) = local_error(x_ref(:,i), x_est(:,i));
% %     u(:,i) = u_ref(:,i) + K*err_loc(:,i);

end

== matlab function Torque_Vectoring_Controller_Controls_2018_Test/CarMaker/Controls/Vehicle Estimated Parameters/Covariantie ==
  data: sensors input; R_beta_lin output; yawrate_lin input; Q_Cy output; car parameter
function [R_beta_lin, Q_Cy] = Covariantie(sensors,yawrate_lin, car)
if (abs(sensors.yawRate)-abs(yawrate_lin)) > car.e_max && abs(sensors.yawRate)>0 && abs(yawrate_lin)>0
    
    global counter
    
    if isempty(counter)
        counter = 0
    end
    
    counter = counter + 1;
    array_dev_yawrate = zeros(1,1.5*(1/car.dt));
    delta = (sensors.wheelAngles(1)+sensors.wheelAngles(2))/2;
    % Q_Cyi wordt hoog gezet, net als R_beta_lin, en hoe groter het verschil, hoe groter de 
    % onnauwkeurigheid zal worden (dev_ya wrate = e uit de paper)
    dev_yawrate = abs(sensors.yawRate)-abs(yawrate_lin);
    
    if counter < 1.5*(1/car.dt)
        array_dev_yawrate(counter) = dev_yawrate;
        
    else
        for k = 2:length(array_dev_yawrate)
            array_dev_yawrate(k-1)=array_dev_yawrate(k);
        end
        array_dev_yawrate(length(array_dev_yawrate)) = dev_yawrate;
    end
    
    dev_yawrate_max = max(array_dev_yawrate);
    % We gaan best een referentiewaarde nemen voor Q_Cyi voor het geval het
    % verschil < car.e_max
    Q_Cy0 = car.Q_Cyref*log(9*(delta/car.delta_max)+1);%functie nog aanpasbaar
    R_beta_lin0 = car.R_beta_linref*log(8*(delta/car.delta_max)+2);
    
    
    
    Q_Cy = Q_Cy0 + 500*dev_yawrate_max^2;
    R_beta_lin = R_beta_lin0 + (5*array_dev_yawrate)^4;
    
else
    delta = (sensors.wheelAngles(1)+sensors.wheelAngles(2))/2;
    Q_Cy0 = car.Q_Cyref*log(9*(delta/car.delta_max)+1);%functie nog aanpasbaar
    R_beta_lin0 = car.R_beta_linref*log(8*(delta/car.delta_max)+2);
    Q_Cy = Q_Cy0;
    R_beta_lin = R_beta_lin0;
end

end

== matlab function Torque_Vectoring_Controller_Controls_2018_Test/CarMaker/Controls/Vehicle Estimated Parameters/Estimation Parameters ==
  data: States input; estimPar output; car parameter; sensors parameter; Fzi input; Fyi input; Fxi input; alpha input; eff input; rref input
function estimPar  = estimation_par(States, car, sensors, Fzi, Fyi, Fxi, alpha, eff, rref)
%% Forming "States_final" %%

estimPar.vy_g = States.vy_g;
estimPar.psi_dot_g = States.psi_dot_g;
estimPar.vx_g = States.vx_g;
estimPar.Cf_g = States.Cf_g;
estimPar.Cr_g = States.Cr_g;
estimPar.Fzi=Fzi;
estimPar.Fxi=Fxi;
estimPar.Fyi=Fyi;
estimPar.alpha_f = alpha.f;
estimPar.alpha_r = alpha.r;
estimPar.eff = eff;
estimPar.rref = rref;
end

== matlab function Torque_Vectoring_Controller_Controls_2018_Test/CarMaker/Controls/Vehicle Estimated Parameters/Fx_estimation ==
  data: States input; Fxi output; car parameter; sensors parameter
function Fxi  = Fx_estimation(States,car, sensors)

%OPM: gearratio zit al verwerkt in sensors.torque (= wheelTorque)

persistent wheelspeedPrev; if isempty(wheelspeedPrev); wheelspeedPrev = [0 ;0 ;0 ;0]; end
persistent inertia; if isempty(inertia); inertia = car.tireInertia; end
if isempty(States.vx_g); States.vx_g =0;end
wheelspeed = sensors.wheelspeed;
alpha = (wheelspeed - wheelspeedPrev)/car.dt;

%wheelTorque = car.gearRatio*sensors.torque -(car.motor.Inertia*car.gearRatio^2 - car.tireInertia)*alpha;
%to be used if only motor torque is known (real scenario)

%Fxi_est = (wheelTorque - alpha*inertia)/car.tireRadius;
Fxi_est = (sensors.torque - alpha*inertia)/car.tireRadius;
%Fxi_est = (sensors.torque)/car.tireRadius;

Fx_tot = sensors.ax*car.mass + 0.5*car.rhoAir*States.vx_g^2*car.Cd*car.AFront;
Fxi = Fxi_est;




wheelspeedPrev=wheelspeed;
inertiaOut = inertia;
end

== matlab function Torque_Vectoring_Controller_Controls_2018_Test/CarMaker/Controls/Vehicle Estimated Parameters/Fy_distribution ==
  data: States input; Fyi output; car parameter; sensors parameter; Fzi input; alpha output
function [Fyi,alpha] = Fy_distribution(States,car, sensors, Fzi)

%% Calculation sideslip angles of the wheels %%
delta = (sensors.wheelAngles(1)+sensors.wheelAngles(2))/2;
alpha.f = -((States.vy_g + car.lf*States.psi_dot_g)/(States.vx_g)) + delta;
alpha.r = -((States.vy_g - car.lr*States.psi_dot_g)/(States.vx_g));

%% Calculation OF Lateral forces (Bycicle model) %%
F_yf = 2*States.Cf_g*alpha.f;
F_yr = 2*States.Cr_g*alpha.r;

%% Distribution of lateral force on left and right tire by using the normal force distribution %%


%Use of a scale factor 

FzRatioFront = [Fzi(1); Fzi(2)]./sum(Fzi(1:2));
FzRatioRear = [Fzi(3); Fzi(4)]./sum(Fzi(3:4));


scaleFactorFy = 0.7;
FyFrontDiff = (FzRatioFront(1) - FzRatioFront(2))*scaleFactorFy/2;
Fy_FL = F_yf/2 + FyFrontDiff* F_yf;
Fy_FR = F_yf/2 - FyFrontDiff* F_yf;
FyRearDiff = (FzRatioRear(1) - FzRatioRear(2))*scaleFactorFy/2;
Fy_RL = F_yr/2 + FyRearDiff* F_yr;
Fy_RR = F_yr/2 - FyRearDiff* F_yr;
    
Fyi=[Fy_FL;Fy_FR;Fy_RL;Fy_RR];

== matlab function Torque_Vectoring_Controller_Controls_2018_Test/CarMaker/Controls/Vehicle Estimated Parameters/Fz_estimation ==
  data: States input; Fzi output; car parameter; sensors parameter
function Fzi  = Fz_estimation(States,car, sensors)

%% Calculation of Normal Forces F_zi %%

if isempty(States.vx_g); States.vx_g =0;end
%Dynamical loads 
%Without taking suspension into account

aero.FD = 0.5*car.Cd*car.AFront*car.rhoAir*States.vx_g^2; %drag force, pointing rearward [N]
aero.FL = 0.5*car.Cl*car.AFront*car.rhoAir*States.vx_g^2; %lift force, pointing upward [N]
aero.lever_FD = [-0.1;0.1]; %distance from the COG to the point of application of the drag [m]
aero.lever_FL = [-0.1;0.1]; %distance from the COG to the point of application of the lift [m]

FFA = car.g*car.mass*car.lr/car.wb - (car.h/car.wb)*(car.mass*sensors.ax) - ...
    aero.FD*((car.h+aero.lever_FD(2))/car.wb) - ...
    aero.FL*((car.lr-aero.lever_FL(1))/car.wb); %dyn load Front Axle
FRA = car.g*car.mass*car.lf/car.wb + (car.h/car.wb)*(car.mass*sensors.ax) + ...
    aero.FD*((car.h+aero.lever_FD(2))/car.wb) - ...
    aero.FL*((car.lf+aero.lever_FL(1))/car.wb); %dyn load Rear Axle


FFL = FFA/2 - (car.h/(2*car.tw))*(car.mass*sensors.ay);
FFR = FFA/2 + (car.h/(2*car.tw))*(car.mass*sensors.ay);
FRL = FRA/2 - (car.h/(2*car.tw))*(car.mass*sensors.ay);
FRR = FRA/2 + (car.h/(2*car.tw))*(car.mass*sensors.ay);


Fzi = [FFL;FFR;FRL;FRR];

== matlab function Torque_Vectoring_Controller_Controls_2018_Test/CarMaker/Controls/Vehicle Estimated Parameters/Efficiency//Power calculation ==
  data: sensors input; eff output; settings input; car parameter; P_elec output; P_mech output; effnotcontrolled output
function [eff,P_elec,P_mech,effnotcontrolled]= Efficiency(sensors,settings,car)
%P_elec * eff = P_mech

persistent effTemp; if isempty(effTemp); effTemp = 0.7; end
persistent errorInt; if isempty(errorInt); errorInt = 0; end

Pmax = car.Pmax - car.PC.safetyMargin; %[W]

P_mech = sum(sensors.torque.*sensors.wheelspeed); %*car.gearRatio
P_elec = sensors.P_elec; if P_elec ==0;P_elec=1;end

ratio = 0.2;


if settings.effEstimation == 1
    
    if P_elec > 1
        effCalc = P_mech/P_elec;
        effTemp = effTemp*ratio + (1-ratio)*min(max(effCalc,car.PC.minEff),car.PC.maxEff);
        
    elseif P_elec < 1
        effCalc = P_elec/min(P_mech,-1);
        effTemp = effTemp*ratio + (1-ratio)*min(max(effCalc,car.PC.minEff),car.PC.maxEff);
        
        
        %mogelijkheid tot uitbreiding: Pmax variable ifv van batterij voor tijdens
        %indurance
    end
    
end

if settings.effEstimation == 2
    
    if P_elec > Pmax*0.3 && sensors.throttle > 0 % only positive power limit
        
        error = (Pmax - P_elec)/Pmax;
        if error < 0 % P_elec > Pmax
            error = error*2;
        end
        
        errorInt = errorInt + error*car.dt;
        errorInt = max(min(errorInt,0.2),-0.2);
        
        dEff = car.PC.Kp*error + car.PC.Ki*errorInt; %more fitting variable name would be powerReductionFactor as this is not anymore an efficiency as Pelec * eff = Pmech
        %make car.PC.Kp velocity dependend?
        
        effTemp = max(min(effTemp + dEff,car.PC.maxEff),car.PC.minEff);
        
    else
        if P_elec > 5000
            eta = P_mech/P_elec;
            effTemp = effTemp*ratio+(1-ratio)*min(max(eta,car.PC.minEff),car.PC.maxEff);
        elseif P_elec < -5000
            eta = P_elec/min(P_mech,-1);
            effTemp = effTemp*ratio+(1-ratio)*min(max(eta,car.PC.minEff),car.PC.maxEff);
        end
        
    end
    
else
    effTemp = effTemp;
    
end


eff = effTemp;
effnotcontrolled = P_mech/P_elec;

== matlab function Torque_Vectoring_Controller_Controls_2018_Test/CarMaker/Controls/Vehicle Estimated Parameters/Slip Ratio ==
  data: States input; slip_ratio output; car parameter; sensors parameter
function slip_ratio = slip_ratio(States, car, sensors)

if isempty(States.vx_g); States.vx_g =0;end
yawRate = [0;0;States.psi_dot_g];
dist = [car.lf   -car.lf   car.lr   -car.lr;
        car.tl/2 -car.tl/2 car.tr/2 -car.tr/2;
        0        0         0        0];
omegaR = sensors.wheelspeed*car.tireRadius;

%Thesis BreyneMeulemans eq 3.20-3.22
v_xcomp = zeros(4,1);
d = sensors.wheelAngles;
for i=1:4
    R = [cos(d(i)) sin(d(i)) 0;
        -sin(d(i)) cos(d(i)) 0;
        0          0         1];
    v_rel = cross(yawRate,dist(:,i));
    v_abs = v_rel + [States.vx_g;0;0];
    v_ab2 = R*v_abs;
    v_xcomp(i) = v_ab2(1);
end

if sensors.ax > 0
    slip_ratio = (omegaR - v_xcomp)./omegaR;
elseif sensors.ax < 0
    slip_ratio = (omegaR - v_xcomp)./v_xcomp;
else
    slip_ratio = [0;0;0;0];
end
end

== matlab function Torque_Vectoring_Controller_Controls_2018_Test/CarMaker/Controls/Vehicle Estimated Parameters/Yawrate Reference ==
  data: rref output; States input; car parameter; sensors parameter
function rref = yawRateRef(States, car, sensors)
if isempty(States.vx_g); States.vx_g =0;end
%Ackermann
wheelAngle = (sensors.wheelAngles(1)+sensors.wheelAngles(2))/2;
rref = wheelAngle*States.vx_g/car.wb;

== matlab function Torque_Vectoring_Controller_Controls_2018_Test/CarMaker/Controls/Vehicle Estimated Parameters/States matrix generator ==
  data: estimPar input; States_matrix_front output; N_est input; Fy_est input; States_matrix_rear output
function [States_matrix_front, States_matrix_rear] = States_matrix_gen(estimPar, N_est, Fy_est)

global counter_mat 

if isempty(counter_mat)
    counter_mat = 0
end

counter_mat = counter_mat+1;
States_matrix_front = zeros(3,1);
States_matrix_rear = zeros(3,1);

while counter_mat < 1000
    States_matrix_front(:,counter_mat) = [estimPar.alpha_f, N_est.f, Fy_est.f];
    States_matrix_rear(:,counter_mat) = [estimPar.alpha_r, N_est.r, Fy_est.r];
    
end
end

== matlab function Torque_Vectoring_Controller_Controls_2018_Test/CarMaker/Controls/Vehicle Estimated Parameters/Normal and lateral force calc ==
  data: States input; N_est output; Fy_est output; car parameter; sensors parameter
function [N_est, Fy_est] = N_F_calc(States, car, sensors)

N_est.f = (car.mass)*9.81*((car.lr)/(car.lr+car.lf))- (sensors.ax)*(car.mass)*(car.h);
N_est.r = (car.mass)*9.81*((car.lr)/(car.lr+car.lf))+ (sensors.ax)*(car.mass)*(car.h);

Fy_est.f = 2*(States.Cf_g)*(alpha.f);
Fy_est.r = 2*(States.Cf_r)*(alpha.r);

== matlab function Torque_Vectoring_Controller_Controls_2018_Test/CarMaker/Controls/Tire model//friction coefficient estimation/Tire model estimation ==
  data: States_matrix_front input; Settings_extended output; States_matrix_rear input; Settings input; Magic_tire_param output
function [Settings_extended, Magic_tire_param] ...
    = Est_tire_model(States_matrix_front, States_matrix_rear, Settings)


if length(States_matrix_front) == 1000   % Indien we sampelen op 100Hz krijgen we dit in 10s
                                         % wat ongeveer de duur is van het
                                         % skidpad event
    p0 = tire_model_est_test(States_matrix_front, States_matrix_rear);
    Settings.act_TV = 1;
end

% The following if-statement is ONLY used when the tire model is
% determined. In the normal case, the driver decides wheter or not he
% activates the TV-mode. When the tire model will be determined (probably
% during skidpad event), following if-statement simply overrules the
% decision of the driver. This means, in the first run of the skidpad
% event, the driver won't be able to use the TV-mode.

if length(States_matrix_front) > 1000
    Settings.torqueMode = 1;
else
    Settings.torqueMode = 0;
end

Settings_extended = Settings;
Magic_tire_param.front_x = p0.front_x;
Magic_tire_param.front_y = p0.front_y;
Magic_tire_param.rear_x = p0.rear_x;
Magic_tire_param.rear_y = p0.rear_y;
